simulink subsystem "Autocode_RT_Pacing"  (R2024b)
settings: Solver=VariableStepAuto  StartTime=0.0  StopTime=10.0  RelTol=1e-3
settings Model: Creator=macheson  LastModifiedBy=macheson

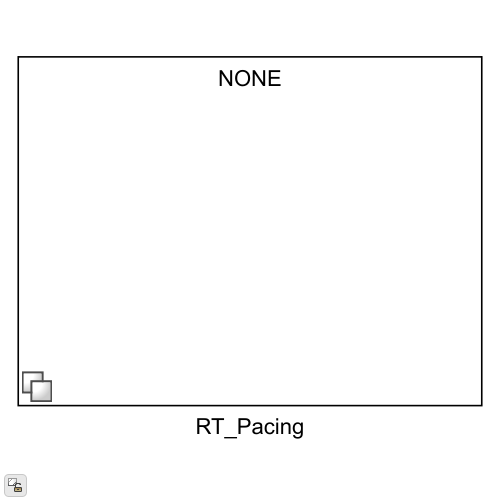
[thumbnail: Simulink's stored preview of the top-level diagram]
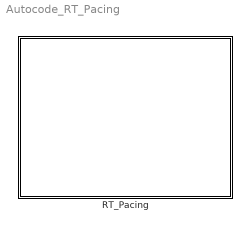
== system Autocode_RT_Pacing ==
  RT_Pacing : Subsystem  Variant=on

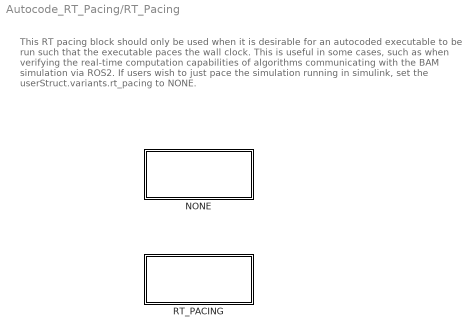
== system Autocode_RT_Pacing/RT_Pacing ==
  note: This RT pacing block should only be used when it is desirable for an autocoded executable to be run such that the executable paces the wall clock. This is useful in some cases, such as when verifying the real-time computation capabilities of algorithms communicating with the BAM simulation via ROS2. If users wish to just pace the simulation running in simulink, set the userStruct.variants.rt_pacing to NONE.
  NONE : Subsystem  VariantControl=RT_TYPE_NONE
  RT_PACING : Subsystem  VariantControl=RT_TYPE_PACE

== system Autocode_RT_Pacing/RT_Pacing/NONE ==

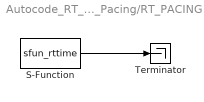
== system Autocode_RT_Pacing/RT_Pacing/RT_PACING ==
  S-Function : S-Function  FunctionName=sfun_rttime  Parameters=1  SFunctionDeploymentMode=off  EnableBusSupport=off
  Terminator : Terminator
  wires:
  S-Function/1 -> Terminator/1
